simulink model "motorsim_SQ"  (R2021a)
settings: Solver=VariableStepAuto  StartTime=0.0  StopTime=10.0  RelTol=1e-3
values from neighbouring files (symbols this model uses):
  b = .5    (= 0.5)    [RunStep_response.m]    (also in Runmotorsim.m)
  J = .05    (= 0.05)    [RunStep_response.m]    (also in Runmotorsim.m)
  Ke = .5    (= 0.5)    [RunStep_response.m]    (also in Runmotorsim.m)
  Kt = 1    [RunStep_response.m]    (also in Runmotorsim.m = 0.5)
  Ra = 1    [RunStep_response.m]    (also in Runmotorsim.m)
settings Model: Creator=Beau Collins  LastModifiedBy=abcollins
settings SolverCC: AlgebraicLoopSolver=TrustRegion
settings DebuggingCC: SFMachineParentedDataDiag=warning

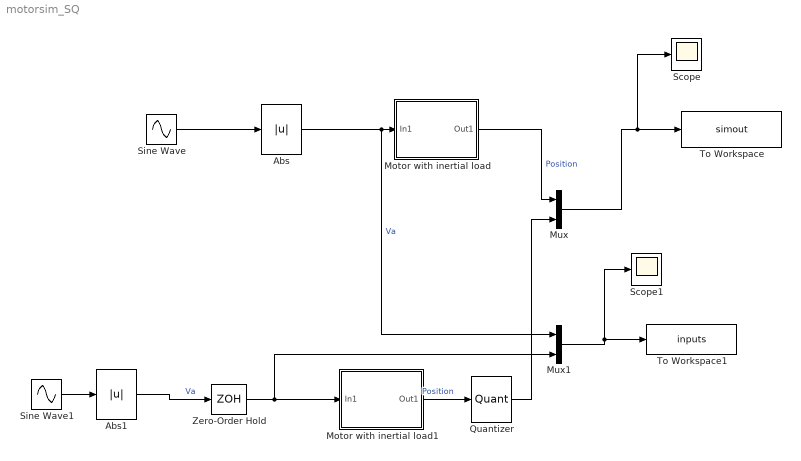
== system motorsim_SQ ==
  Abs : Abs
  Abs1 : Abs
  Motor with inertial load : Subsystem
  Motor with inertial load1 : Subsystem
  Mux : Mux  Inputs=2
  Mux1 : Mux  Inputs=2
  Quantizer : Quantizer
  Scope : Scope
  Scope1 : Scope
  Sine Wave : Sin  SampleTime=0
  Sine Wave1 : Sin  SampleTime=0
  To Workspace : ToWorkspace  VariableName=simout  SaveFormat=Timeseries  SampleTime=-1
  To Workspace1 : ToWorkspace  VariableName=inputs  SaveFormat=Timeseries  SampleTime=-1
  Zero-Order Hold : ZeroOrderHold  SampleTime=-1
  wires:
  Sine Wave/1 -> Abs/1
  Abs/1 -> Mux1/1, Motor with inertial load/1(In1)  "Va"
  Motor with inertial load/1(Out1) -> Mux/1  "Position"
  Sine Wave1/1 -> Abs1/1
  Abs1/1 -> Zero-Order Hold/1  "Va"
  Mux/1 -> Scope/1, To Workspace/1
  Mux1/1 -> Scope1/1, To Workspace1/1
  Motor with inertial load1/1(Out1) -> Quantizer/1  "Position"
  Quantizer/1 -> Mux/2
  Zero-Order Hold/1 -> Mux1/2, Motor with inertial load1/1(In1)

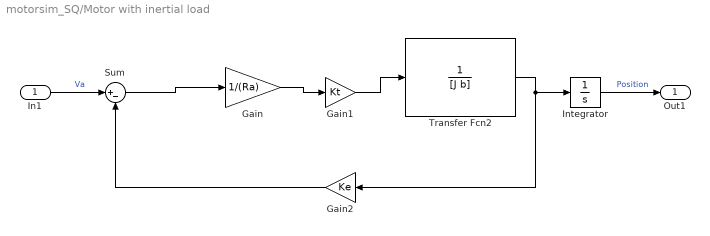
== system motorsim_SQ/Motor with inertial load ==
  In1 : Inport
  Gain : Gain  Gain=1/(Ra)
  Gain1 : Gain  Gain=Kt
  Gain2 : Gain  Gain=Ke
  Integrator : Integrator
  Sum : Sum  Inputs=|+-
  Transfer Fcn2 : TransferFcn  Denominator=[J b]  ContinuousStateAttributes='Transfer_Fcn'
  Out1 : Outport
  wires:
  In1/1 -> Sum/1  "Va"
  Transfer Fcn2/1 -> Gain2/1, Integrator/1
  Sum/1 -> Gain/1
  Gain2/1 -> Sum/2
  Gain/1 -> Gain1/1
  Integrator/1 -> Out1/1  "Position"
  Gain1/1 -> Transfer Fcn2/1

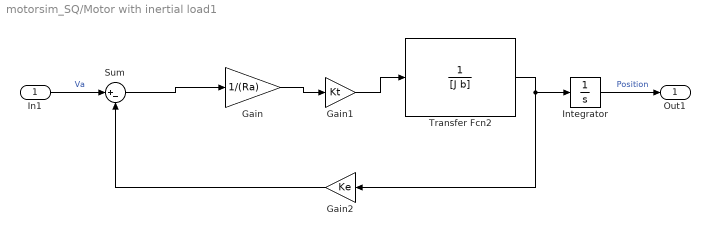
== system motorsim_SQ/Motor with inertial load1 ==
  In1 : Inport
  Gain : Gain  Gain=1/(Ra)
  Gain1 : Gain  Gain=Kt
  Gain2 : Gain  Gain=Ke
  Integrator : Integrator
  Sum : Sum  Inputs=|+-
  Transfer Fcn2 : TransferFcn  Denominator=[J b]  ContinuousStateAttributes='Transfer_Fcn'
  Out1 : Outport
  wires:
  In1/1 -> Sum/1  "Va"
  Transfer Fcn2/1 -> Gain2/1, Integrator/1
  Sum/1 -> Gain/1
  Gain2/1 -> Sum/2
  Gain/1 -> Gain1/1
  Integrator/1 -> Out1/1  "Position"
  Gain1/1 -> Transfer Fcn2/1
